simulink model "exercise3_sl"  (R2019b)
settings: Solver=FixedStepAuto  StartTime=0.0  StopTime=10  FixedStep=1e-3  RelTol=1e-3  EnableMultiTasking=on
settings Model: ExtModeTrigMode=oneshot  ExtModeArmWhenConnect=off  Creator=lucam  LastModifiedBy=lucam
settings DataIOCC: SaveFormat=Array  SignalLoggingSaveFormat=ModelDataLogs  ReturnWorkspaceOutputs=off
settings OptimizationCC: BlockReduction=off  BooleanDataType=off
settings DebuggingCC: SaveWithParameterizedLinksMsg=none  UnderspecifiedInitializationDetection=Classic  MergeDetectMultiDrivingBlocksExec=none  SignalResolutionControl=TryResolveAllWithWarning  MultiTaskDSMMsg=warning  MultiTaskCondExecSysMsg=none  ArithmeticOperatorsInVariantConditions=warning
settings HardwareCC: TargetUnknown=on
settings ModelReferenceCC: PropagateSignalLabelsOutOfModel=off
settings SFSimCC: SimUseLocalCustomCode=off  CustomCodeUndefinedFunction=UseInterfaceOnly
settings RTWCC: RTWUseLocalCustomCode=off
settings GRTTargetCC: TargetLangStandard=C89/C90 (ANSI)  CombineOutputUpdateFcns=off  GRTInterface=on

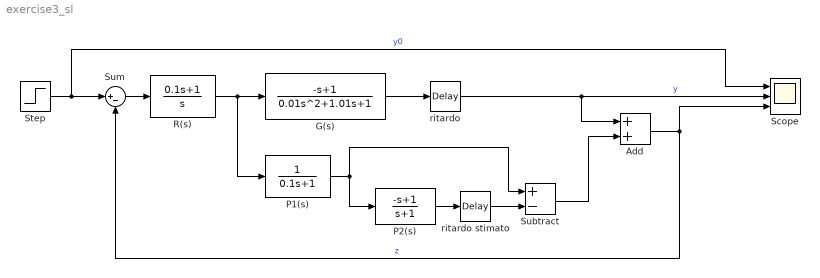
== system exercise3_sl ==
  Add : Sum
  G(s) : TransferFcn  Numerator=[-1 1]  Denominator=[0.01 1.01 1]
  P1(s) : TransferFcn  Numerator=1  Denominator=[0.1 1]
  P2(s) : TransferFcn  Numerator=[-1 1]  Denominator=[1 1]
  R(s) : TransferFcn  Numerator=[0.1 1]  Denominator=[1 0]
  Scope : Scope  NumInputPorts=3
  Step : Step  Time=0  SampleTime=0
  Subtract : Sum  Inputs=+-
  Sum : Sum  Inputs=|+-  SaturateOnIntegerOverflow=on  InputSameDT=on  OutDataTypeStr=Inherit: Same as first input
  ritardo : TransportDelay
  ritardo stimato : TransportDelay
  wires:
  Sum/1 -> R(s)/1
  G(s)/1 -> ritardo/1
  P2(s)/1 -> ritardo stimato/1
  ritardo stimato/1 -> Subtract/2
  P1(s)/1 -> Subtract/1, P2(s)/1
  Add/1 -> Scope/3, Sum/2  "z"
  R(s)/1 -> G(s)/1, P1(s)/1
  Step/1 -> Scope/1, Sum/1  "y0"
  Subtract/1 -> Add/2
  ritardo/1 -> Scope/2, Add/1  "y"
